simulink model "ReceiverLowIF"  (R2021a)
settings: Solver=VariableStepAuto  StartTime=0.0  StopTime=10.0  RelTol=1e-3
undefined symbols (not defined in the file or in its folder): physconst, S
libraries: simrfV2elements x3, simrfV2util1 x3, simrfV2systems x1, simrfV2sources1 x1
settings Model: Creator=gzucchel  LastModifiedBy=gzucchel
settings DataIOCC: ExternalInput=externalInput_tp2a668ad5_623b_4b0a_a91a_a9b0c995a288  InitialState=initialState_tp2a668ad5_623b_4b0a_a91a_a9b0c995a288  LoadExternalInput=on  LoadInitialState=on  SaveFinalState=on  SaveOperatingPoint=on  SaveFormat=Structure

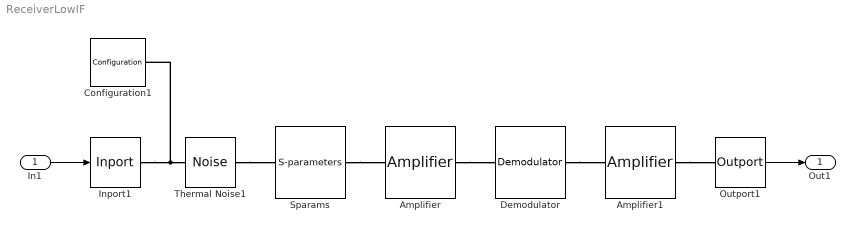
== system ReceiverLowIF ==
  In1 : Inport  PortDimensions=2  SampleTime=2e-08  Interpolate=off
      settings: SignalType=complex
  Amplifier : simrfV2elements/Amplifier  classname=amplifier  DataSource=Data file  File=unitygain.s2p  Paramtype=S-parameters  Sparam=[0 0;1 0]  SparamFreq=1e9 Hz  SparamZ0=50  Residues=0  Poles=0  DF={0 0; 1 0}  Source_linear_gain=Available power gain  linear_gain=18 dB  Zin=50  Zout=50  Source_Poly=Even and odd order  Poly_Coeffs=[0 1]  IPType=Output  IP2=Inf dBm  IP3=23 dBm  P1dB=inf dBm  Psat=inf dBm  Gcomp=inf dBm  InternalGrounding=on  SourceFreq=Extracted from data source  PlotFreq=[1e9:1e6:3e9] Hz  PlotType=X-Y plane  YParam1=S(1,1)  YFormat1=Magnitude (decibels)  YParam2=None  YFormat2=Magnitude (decibels)  YOption=Linear  XOption=Linear  SparamRepresentation=Time domain (rationalfit)  FitTol=-40  FitOpt=Fit individually  AutoImpulseLength=on  ImpulseLength=1e-10 s  MagModeling=off  AddNoise=on  NoiseType=Noise figure  NoiseDist=White  NF=2.1  MinNF=0  Gopt=0  RN=0  CarrierFreq=0 Hz  NoiseAutoImpulseLength=on  NoiseImpulseLength=1e-10 s  SpecifyOpFreq=off  OpFreq=0 Hz
      settings: SourceProductBaseCode=RB
  Amplifier1 : simrfV2elements/Amplifier  classname=amplifier  DataSource=Data file  File=unitygain.s2p  Paramtype=S-parameters  Sparam=[0 0;1 0]  SparamFreq=1e9 Hz  SparamZ0=50  Residues=0  Poles=0  DF={0 0; 1 0}  Source_linear_gain=Available power gain  linear_gain=15 dB  Zin=50  Zout=50  Source_Poly=Even and odd order  Poly_Coeffs=[0 1]  IPType=Output  IP2=54 dBm  IP3=36 dBm  P1dB=inf dBm  Psat=inf dBm  Gcomp=inf dBm  InternalGrounding=on  SourceFreq=Extracted from data source  PlotFreq=[1e9:1e6:3e9] Hz  PlotType=X-Y plane  YParam1=S(1,1)  YFormat1=Magnitude (decibels)  YParam2=None  YFormat2=Magnitude (decibels)  YOption=Linear  XOption=Linear  SparamRepresentation=Time domain (rationalfit)  FitTol=-40  FitOpt=Fit individually  AutoImpulseLength=on  ImpulseLength=1e-10 s  MagModeling=off  AddNoise=on  NoiseType=Noise figure  NoiseDist=White  NF=4  MinNF=0  Gopt=0  RN=0  CarrierFreq=0 Hz  NoiseAutoImpulseLength=on  NoiseImpulseLength=1e-10 s  SpecifyOpFreq=off  OpFreq=0 Hz
      settings: SourceProductBaseCode=RB
  Configuration1 : simrfV2util1/Configuration  AutoFreq=off  Tones=[0.05 2.4] GHz  Harmonics=[3 1]  NormalizeCarrierPower=on  SolverType=Auto  UseCCode=on  StepSize=2e-08 s  AddNoise=on  defaultRNG=on  Seed=0  Temperature=290.0 K  SolverDelFlag=0  AbsTol=1e-6  RelTol=1e-3  MaxIter=10  ErrorEstimationType=2-norm over all variables  EnableInterpFilter=on  HiddenFIRfilterControllerParam=on  SmallSignalApprox=off  AllSimFreqs=on  SimFreqs=[] Hz  SimFreqsInternal=[]  SamplesPerFrame=1
      settings: SourceProductBaseCode=RB
  Demodulator : simrfV2systems/Demodulator  classname=rfdemod  Source_linear_gain=Available power gain  linear_gain=-6 dB  Poly_Coeffs=[0 1]  LOFreq=2.45 GHz  Zin=50  Zout=50  AddIRFilter=off  AddCSFilter=on  InternalGrounding=on  ForceNextInit=off  Source_Poly=Even and odd order  IPType=Output  IP2=Inf dBm  IP3=33 dBm  P1dB=inf dBm  Psat=inf dBm  Gcomp=inf dBm  NF=5.4  Isolation=inf dB  AddPhaseNoise=off  PhaseNoiseOffset=1  PhaseNoiseLevel=-Inf  AutoImpulseLengthPN=on  ImpulseLengthPN=1e-10  ImpulseLength_unitPN=s  DesignMethodIR=Ideal  ResponseTypeIR=Highpass  ImplementationIR=LC Tee  ImplementationIdealIR=Constant per carrier  ImplementationRationalIR=Transfer function  UseFilterOrderIR=on  FilterOrderIR=3  PassFreq_lpIR=2.4005  PassFreq_lp_unitIR=GHz  PassFreq_hpIR=2.3995  PassFreq_hp_unitIR=GHz  PassFreq_bpIR=[2.3995 2.4005]  PassFreq_bp_unitIR=GHz  PassFreq_bsIR=[2.499499999 2.500500001]  PassFreq_bs_unitIR=GHz  PassAttenIR=10*log10(2)  StopFreq_lpIR=2.400500001  StopFreq_lp_unitIR=GHz  StopFreq_hpIR=2.399499999  StopFreq_hp_unitIR=GHz  StopFreq_bpIR=[2.399499999 2.400500001]  StopFreq_bp_unitIR=GHz  StopFreq_bsIR=[2.4995 2.5005]  StopFreq_bs_unitIR=GHz  StopAttenIR=40  RsrcIR=50  RloadIR=50  AutoImpulseLengthIR=on  ImpulseLengthIR=1e-10  ImpulseLength_unitIR=s  DesignMethodCS=Ideal  ResponseTypeCS=Lowpass  ImplementationCS=LC Tee  ImplementationIdealCS=Constant per carrier  ImplementationRationalCS=Transfer function  UseFilterOrderCS=on  FilterOrderCS=3  PassFreq_lpCS=50.5  PassFreq_lp_unitCS=MHz  PassFreq_hpCS=49.5  PassFreq_hp_unitCS=MHz  PassFreq_bpCS=[49.5 50.5]  PassFreq_bp_unitCS=MHz  PassFreq_bsCS=[4.849499999 4.850500001]  PassFreq_bs_unitCS=GHz  PassAttenCS=10*log10(2)  StopFreq_lpCS=50.500001  StopFreq_lp_unitCS=MHz  StopFreq_hpCS=49.499999  StopFreq_hp_unitCS=MHz  StopFreq_bpCS=[49.499999 50.500001]  StopFreq_bp_unitCS=MHz  StopFreq_bsCS=[4.8495 4.8505]  StopFreq_bs_unitCS=GHz  StopAttenCS=40  RsrcCS=50  RloadCS=50  AutoImpulseLengthCS=on  ImpulseLengthCS=1e-10  ImpulseLength_unitCS=s
      settings: SourceProductBaseCode=RB
  Inport1 : simrfV2util1/Inport  SimulinkInputSignalType=Power  CarrierFreq=[2.4 2.5] GHz  ZS=50  InternalGrounding=on
      settings: SourceProductBaseCode=RB
  Outport1 : simrfV2util1/Outport  SensorType=Power  OutputFormat=Complex Baseband  CarrierFreq=[50] MHz  ZL=50  InternalGrounding=on  StepSize=1e-6 s  AutoStep=on
      settings: SourceProductBaseCode=RB
  Sparams : simrfV2elements/S-parameters  classname=sparam_element  DataSource=Data file  File=Passive_filter.s2p  Paramtype=S-parameters  Sparam=[0 0;1 0]  SparamFreq=1e9 Hz  SparamZ0=50  Residues=0  Poles=0  DF={0 0; 1 0}  FitOpt=Share all poles  FitTol=-40  SourceFreq=Extracted from data source  PlotFreq=[1e9:1e6:3e9] Hz  PlotType=X-Y plane  YParam1=S(2,1)  YFormat1=Magnitude (decibels)  YParam2=None  YFormat2=Magnitude (decibels)  YOption=Linear  XOption=Linear  AddNoise=on  InternalGrounding=on  SparamRepresentation=Time domain (rationalfit)  AutoImpulseLength=on  ImpulseLength=1e-10 s  MagModeling=off  CacheLevel=0
      settings: SourceProductBaseCode=RB
  Thermal Noise1 : simrfV2sources1/Noise  SimulinkInputSignalType=Ideal voltage  NoiseType=White  NoisePSD=4*physconst('Boltzmann')*290*50  CarrierFreq=0 Hz  AutoImpulseLength=on  ImpulseLength=1e-10 s  InternalGrounding=off
      settings: SourceProductBaseCode=RB
  Out1 : Outport  PortDimensions=1  SampleTime=2e-08
  wires:
  In1/1 -> Inport1/1
  Outport1/1 -> Out1/1
  connections:
  Configuration1/LConn1 -- Inport1/RConn1 -- Thermal Noise1/RConn1
  Thermal Noise1/LConn1 -- Sparams/LConn1
  Sparams/RConn1 -- Amplifier/LConn1
  Amplifier/RConn1 -- Demodulator/LConn1
  Demodulator/RConn1 -- Amplifier1/LConn1
  Amplifier1/RConn1 -- Outport1/LConn1
